simulink model "test_RF"  (R2023a)
settings: Solver=FixedStepAuto  StartTime=0.0  StopTime=inf  RelTol=1e-3  EnableMultiTasking=on
libraries: px4Sensorslib x1
settings Model: SimulationMode=external  ExtModeTrigDuration=10  Creator=ArriGE66  LastModifiedBy=ArriGE66
settings SolverCC: PositivePriorityOrder=on
settings OptimizationCC: EnhancedBackFolding=on  PassReuseOutputArgsAs=Individual arguments  ZeroExternalMemoryAtStartup=off  ZeroInternalMemoryAtStartup=off  MaxStackSize=64  OptimizeBlockOrder=speed  DifferentSizesBufferReuse=on  OptimizationCustomize=off  EfficientTunableParamExpr=on
settings DebuggingCC: ParameterTunabilityLossMsg=error
settings HardwareCC: ProdBitPerPointer=32  ProdBitPerSizeT=32  ProdBitPerPtrDiffT=32  ProdLargestAtomicInteger=Long  ProdLargestAtomicFloat=Double  ProdWordSize=32  ProdLongLongMode=on  ProdHWDeviceType=ARM Compatible->ARM Cortex
settings SFSimCC: MATLABDynamicMemAlloc=off  SimTargetLang=C++
settings RTWCC: Description=Embedded Coder  SystemTargetFile=ert.tlc  HardwareBoard=PX4 Cube Orange  TemplateMakefile=ert_default_tmf  Toolchain=GNU Tools for PX4 Autopilots  TargetLang=C++
settings CodeAppCC: ForceParamTrailComments=on  IgnoreCustomStorageClasses=off  OperatorAnnotations=on  SimulinkDataObjDesc=on  SFDataObjDesc=on  InsertBlockDesc=on
settings ERTTargetCC: ExtMode=on  ExtModeTransport=3  ExtModeStaticAlloc=on  ExtModeStaticAllocSize=1024  ExtModeMexFile=ext_xcp  ExtModeMexArgs=1 COM10 3000000  ExtModeIntrfLevel=Level2 - Open

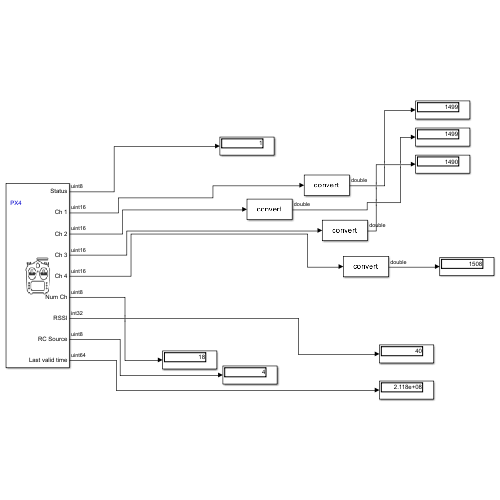
[thumbnail: Simulink's stored preview of the top-level diagram]
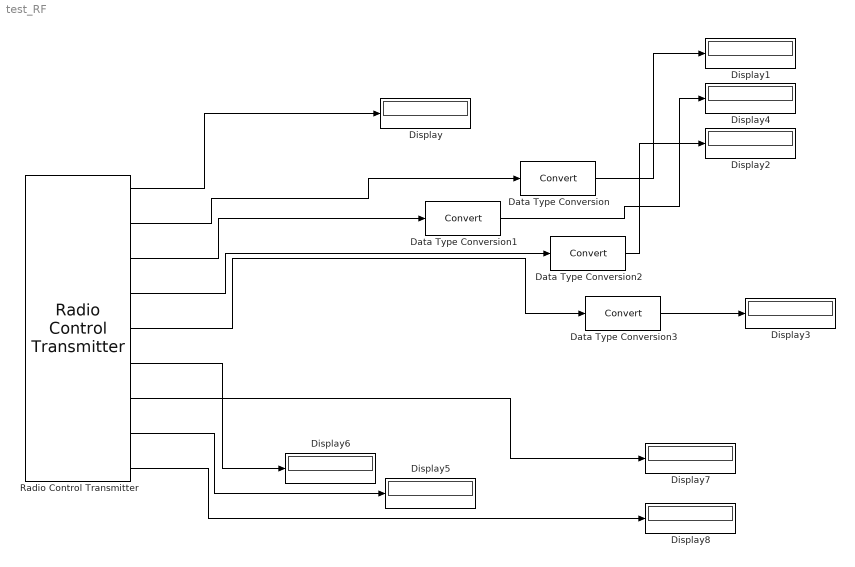
== system test_RF ==
  Data Type Conversion{,1..3} (4 alike) : DataTypeConversion  SaturateOnIntegerOverflow=off  RndMeth=Floor
  Display{,1..8} (9 alike) : Display
  Radio Control Transmitter : px4Sensorslib/Radio Control Transmitter  channel1=on  channel2=on  channel3=on  channel4=on  channel5=off  channel6=off  channel7=off  channel8=off  channel_count=on  rssi=on  rc_input_source=on  timestamp_last_signal=on  time_stamp=off  sampleTime=1/250  BlockingMode=off  BlockTimeout=5
  wires:
  Radio Control Transmitter/1 -> Display/1
  Radio Control Transmitter/5 -> Data Type Conversion3/1
  Radio Control Transmitter/4 -> Data Type Conversion2/1
  Radio Control Transmitter/8 -> Display5/1
  Radio Control Transmitter/6 -> Display6/1
  Radio Control Transmitter/7 -> Display7/1
  Radio Control Transmitter/9 -> Display8/1
  Radio Control Transmitter/2 -> Data Type Conversion/1
  Data Type Conversion/1 -> Display1/1
  Data Type Conversion2/1 -> Display2/1
  Radio Control Transmitter/3 -> Data Type Conversion1/1
  Data Type Conversion1/1 -> Display4/1
  Data Type Conversion3/1 -> Display3/1
